simulink model "Linear_Simulation_CTC_Circle"  (R2020a)
settings: Solver=ode4  StartTime=0.0  StopTime=50  FixedStep=1e-3  RelTol=1e-3
undefined symbols (not defined in the file): Actc, Bctc, Cctc, K, xs0
settings Model: Creator=Pere Giró  LastModifiedBy=Pere Giró

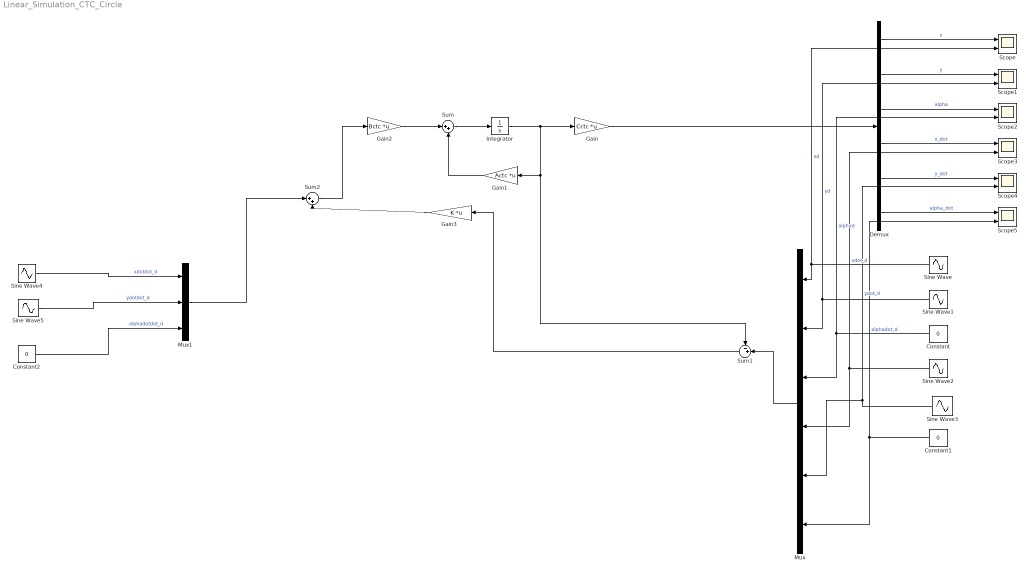
== system Linear_Simulation_CTC_Circle ==
  Constant : Constant  Value=0
  Constant1 : Constant  Value=0
  Constant2 : Constant  Value=0
  Demux : Demux  Outputs=6
  Gain : Gain  Gain=Cctc  Multiplication=Matrix(K*u)
  Gain1 : Gain  Gain=Actc  Multiplication=Matrix(K*u)
  Gain2 : Gain  Gain=Bctc  Multiplication=Matrix(K*u)
  Gain3 : Gain  Gain=K  Multiplication=Matrix(K*u)
  Integrator : Integrator  InitialCondition=xs0
  Mux : Mux  Inputs=6
  Mux1 : Mux  Inputs=3
  Scope{,1..5} (6 alike) : Scope  NumInputPorts=2
  Sine Wave : Sin  Frequency=0.3  SampleTime=0
  Sine Wave1 : Sin  Bias=-1  Frequency=0.3  Phase=pi/2  SampleTime=0
  Sine Wave2 : Sin  Amplitude=0.3  Frequency=0.3  Phase=pi/2  SampleTime=0
  Sine Wave3 : Sin  Amplitude=-0.3  Frequency=0.3  SampleTime=0
  Sine Wave4 : Sin  Amplitude=-0.3^2  Frequency=0.3  SampleTime=0
  Sine Wave5 : Sin  Amplitude=-0.3^2  Frequency=0.3  Phase=pi/2  SampleTime=0
  Sum : Sum  Inputs=|++
  Sum1 : Sum  Inputs=-+|
  Sum2 : Sum  Inputs=|++
  wires:
  Gain2/1 -> Sum/1
  Gain1/1 -> Sum/2
  Sum/1 -> Integrator/1
  Integrator/1 -> Gain1/1, Sum1/1, Gain/1
  Gain/1 -> Demux/1
  Demux/1 -> Scope/1  "x"
  Demux/2 -> Scope1/1  "y"
  Demux/3 -> Scope2/1  "alpha"
  Demux/4 -> Scope3/1  "x_dot"
  Demux/5 -> Scope4/1  "y_dot"
  Demux/6 -> Scope5/1  "alpha_dot"
  Sum1/1 -> Gain3/1
  Mux/1 -> Sum1/2
  Sine Wave1/1 -> Scope1/2, Mux/2  "yd"
  Sine Wave/1 -> Scope/2, Mux/1  "xd"
  Constant/1 -> Scope2/2, Mux/3  "alphad"
  Sine Wave2/1 -> Scope3/2, Mux/4  "xdot_d"
  Sine Wave3/1 -> Scope4/2, Mux/5  "ydot_d"
  Constant1/1 -> Scope5/2, Mux/6  "alphadot_d"
  Constant2/1 -> Mux1/3  "alphadotdot_d"
  Sine Wave4/1 -> Mux1/1  "xdotdot_d"
  Sine Wave5/1 -> Mux1/2  "ydotdot_d"
  Gain3/1 -> Sum2/2
  Sum2/1 -> Gain2/1
  Mux1/1 -> Sum2/1
